simulink model "pid_test3"  (Simulink 6.1)
settings: Solver=ode3  StartTime=0.0  StopTime=40  FixedStep=0.01  RelTol=1e-3
libraries: simulink x1
settings Model: LastModifiedBy=murahasi
settings DebuggingCC: SolverPrmCheckMsg=warning

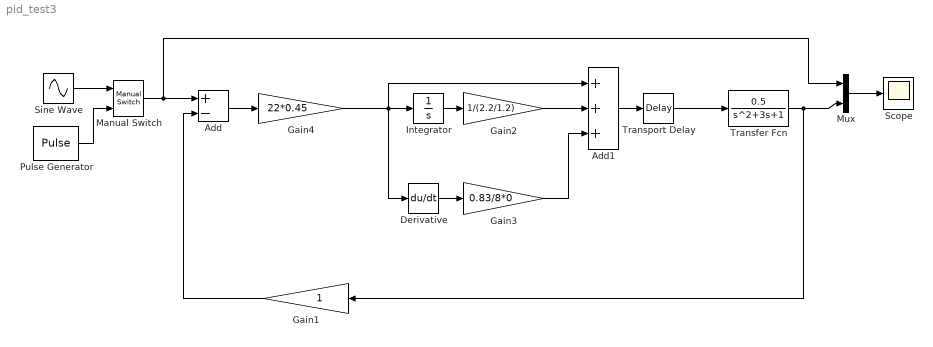
== system pid_test3 ==
  Add : Sum  Inputs=+-  OutScaling=2^-10
  Add1 : Sum  Inputs=+++  OutScaling=2^-10
  Derivative : Derivative
  Gain1 : Gain  Orientation=left
  Gain2 : Gain  Gain=1/(2.2/1.2)
  Gain3 : Gain  Gain=0.83/8*0
  Gain4 : Gain  Gain=22*0.45
  Integrator : Integrator
  Manual Switch : simulink/Signal Routing/Manual Switch  sw=0  action=0
  Mux : Mux  Inputs=2
  Pulse Generator : DiscretePulseGenerator  PulseType=Time based  Period=10  PulseWidth=50
  Scope : Scope
  Sine Wave : Sin  Frequency=2*pi*1  SampleTime=0
  Transfer Fcn : TransferFcn  Numerator=[0.5]  Denominator=[1 3 1]
  Transport Delay : TransportDelay  DelayTime=0.3
  wires:
  Add1/1 -> Transport Delay/1
  Add/1 -> Gain4/1
  Manual Switch/1 -> Add/1, Mux/1
  Transfer Fcn/1 -> Mux/2, Gain1/1
  Mux/1 -> Scope/1
  Sine Wave/1 -> Manual Switch/1
  Pulse Generator/1 -> Manual Switch/2
  Integrator/1 -> Gain2/1
  Gain2/1 -> Add1/2
  Derivative/1 -> Gain3/1
  Gain3/1 -> Add1/3
  Gain4/1 -> Integrator/1, Derivative/1, Add1/1
  Gain1/1 -> Add/2
  Transport Delay/1 -> Transfer Fcn/1
